simulink model "NonLinearMF"  (R2017a)
settings: Solver=ode5  StartTime=0.0  StopTime=30  FixedStep=0.01  RelTol=1e-3
values from neighbouring files (symbols this model uses):
  b10 = 6.05e-3    (= 0.00605)    [FurutaConstants.m]
  b20 = 5.52e-04    (= 0.000552)    [FurutaConstants.m]
  g0 = 9.81    [FurutaConstants.m]
  I1z0 = 3.7365e-3    (= 0.0037365)    [FurutaConstants.m]
  I2x0 = 0.2927e-3    (= 0.0002927)    [FurutaConstants.m]
  I2y0 = 0.2937e-3    (= 0.0002937)    [FurutaConstants.m]
  I2z0 = 0.0051e-3    (= 5.1e-06)    [FurutaConstants.m]
  Ixz20 = -0.0131e-3    (= -1.31e-05)    [FurutaConstants.m]
  K = [0 0 0 1]*(inv(M))*Phi    [Ackermanns.m]    (also in FurutaConstants.m = place(A,B,poles1))
  kt0 = 0.122326    [FurutaConstants.m]
  L10 = 230.45e-3    (= 0.23045)    [FurutaConstants.m]
  l10 = -56.69e-3    (= -0.05669)    [FurutaConstants.m]
  l20 = 58.18e-3    (= 0.05818)    [FurutaConstants.m]
  m10 = 0.36233    [FurutaConstants.m]
  m20 = 0.04948    [FurutaConstants.m]
  Rm0 = 12.38    [FurutaConstants.m]
  theta1o = 0    [FurutaConstants.m]
  theta2o = 14*pi/180    (= 0.244346095279)    [FurutaConstants.m]
settings Model: Creator=felip  LastModifiedBy=felip

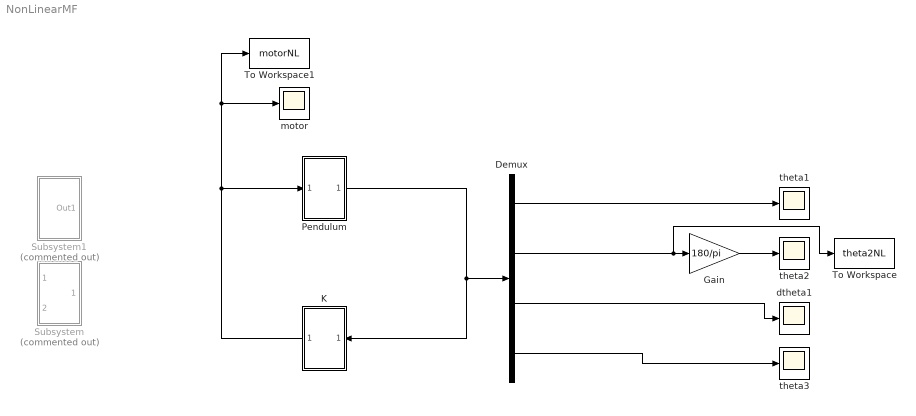
== system NonLinearMF ==
  Demux : Demux
  Gain : Gain  Gain=180/pi
  K : Subsystem
  Pendulum : Subsystem
  Subsystem : Subsystem  Commented=on
  Subsystem1 : Subsystem  Commented=on
  To Workspace : ToWorkspace  VariableName=theta2NL  SaveFormat=Timeseries  SampleTime=-1
  To Workspace1 : ToWorkspace  VariableName=motorNL  SaveFormat=Timeseries  SampleTime=-1
  dtheta1 : Scope
  "motor " : Scope
  theta1 : Scope
  theta2 : Scope
  theta3 : Scope
  wires:
  Pendulum/1(Out1) -> K/1(In1), Demux/1
  Demux/2 -> To Workspace/1, Gain/1
  Demux/1 -> theta1/1
  Demux/3 -> dtheta1/1
  Gain/1 -> theta2/1
  Demux/4 -> theta3/1
  K/1(Out1) -> Pendulum/1(In1), "motor "/1, To Workspace1/1

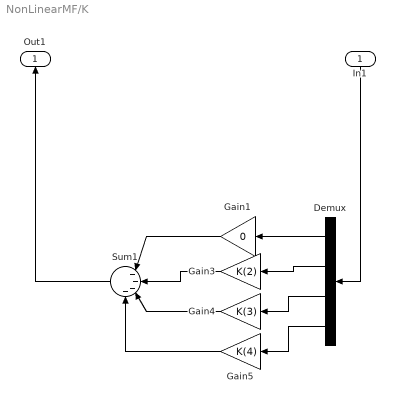
== system NonLinearMF/K ==
  In1 : Inport
  Demux : Demux
  Gain1 : Gain  Gain=0
  Gain3 : Gain  Gain=K(2)
  Gain4 : Gain  Gain=K(3)
  Gain5 : Gain  Gain=K(4)
  Sum1 : Sum  Inputs=|----
  Out1 : Outport
  wires:
  Demux/2 -> Gain3/1
  Demux/4 -> Gain5/1
  In1/1 -> Demux/1
  Gain4/1 -> Sum1/3
  Demux/3 -> Gain4/1
  Gain1/1 -> Sum1/1
  Gain5/1 -> Sum1/4
  Demux/1 -> Gain1/1
  Sum1/1 -> Out1/1
  Gain3/1 -> Sum1/2

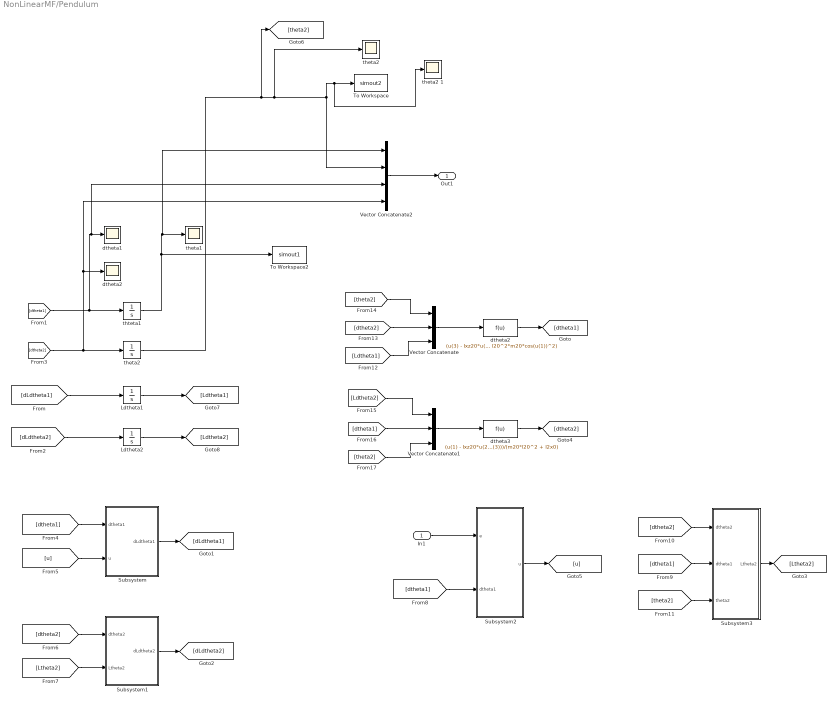
== system NonLinearMF/Pendulum ==
  In1 : Inport
  Ldtheta1 : Integrator
  Ldtheta2 : Integrator
  Subsystem : Subsystem
  Subsystem1 : Subsystem
  Subsystem2 : Subsystem
  Subsystem3 : Subsystem
  To Workspace : ToWorkspace  VariableName=simout2  SaveFormat=Timeseries  SampleTime=-1
  To Workspace2 : ToWorkspace  VariableName=simout1  SaveFormat=Timeseries  SampleTime=-1
  Vector Concatenate : Concatenate  NumInputs=3
  Vector Concatenate1 : Concatenate  NumInputs=3
  Vector Concatenate2 : Concatenate  NumInputs=4
  dtheta1 : Scope
  dtheta2 : Fcn  Expr=(u(3) - Ixz20*u(2)*cos(u(1)) + L10*u(2)*l20*m20*cos(u(1)))/(I2y0 + I1z0 + L10^2*m20 + l10^2*m10 + l20^2*m20 - I2y0*cos(u(1))^2 + I2z0*cos(u(1))^2 - l20^2*m20*cos(u(1))^2)
  "dtheta2 " : Scope
  dtheta3 : Fcn  Expr=(u(1) - Ixz20*u(2)*cos(u(3)) + L10*u(2)*l20*m20*cos(u(3)))/(m20*l20^2 + I2x0)
  theta1 : Scope
  theta2 : Integrator  InitialCondition=theta2o
  "theta2 " : Scope
  theta2 1 : Scope
  thteta1 : Integrator  InitialCondition=theta1o
  Out1 : Outport
  wires:
  In1/1 -> Subsystem2/1(e)
  Vector Concatenate2/1 -> Out1/1
  dtheta2/1 -> [dtheta1]
  [dtheta1] -> thteta1/1, Vector Concatenate2/3, dtheta1/1
  Subsystem1/1(dLdtheta2) -> [dLdtheta2]
  Vector Concatenate1/1 -> dtheta3/1
  [Ltheta2] -> Subsystem1/2(Ltheta2)
  Vector Concatenate/1 -> dtheta2/1
  [dtheta2] -> Vector Concatenate2/4, "dtheta2 "/1, theta2/1
  [dtheta1] -> Subsystem2/2(dtheta1)
  [theta2] -> Vector Concatenate1/3
  [dtheta2] -> Vector Concatenate/2
  [dLdtheta2] -> Ldtheta2/1
  [dLdtheta1] -> Ldtheta1/1
  Subsystem3/1("Ltheta2 ") -> [Ltheta2]
  Ldtheta1/1 -> [Ldtheta1]
  [theta2] -> Vector Concatenate/1
  Subsystem/1(dLdtheta1) -> [dLdtheta1]
  Ldtheta2/1 -> [Ldtheta2]
  [Ldtheta2] -> Vector Concatenate1/1
  thteta1/1 -> Vector Concatenate2/1, theta1/1, To Workspace2/1
  [dtheta1] -> Subsystem/1(dtheta1)
  [dtheta2] -> Subsystem1/1(dtheta2)
  Subsystem2/1("u ") -> [u]
  [theta2] -> Subsystem3/3(theta2)
  [dtheta1] -> Vector Concatenate1/2
  [dtheta1] -> Subsystem3/2(dtheta1)
  [Ldtheta1] -> Vector Concatenate/3
  [u] -> Subsystem/2(u)
  [dtheta2] -> Subsystem3/1(dtheta2)
  theta2/1 -> [theta2], Vector Concatenate2/2, theta2 1/1, To Workspace/1, "theta2 "/1
  dtheta3/1 -> [dtheta2]

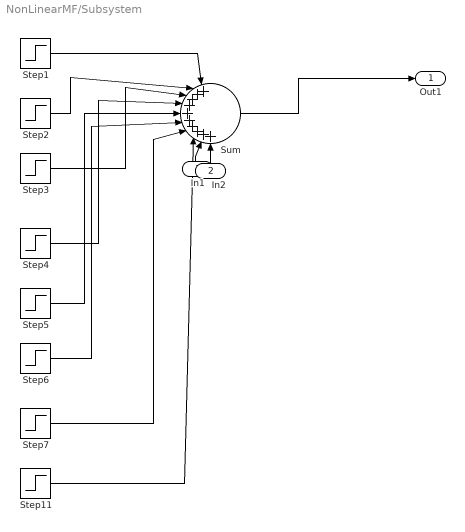
== system NonLinearMF/Subsystem ==
  In1 : Inport
  In2 : Inport  Port=2
  Step1 : Step  Time=10  After=12  SampleTime=0
  Step11 : Step  Time=14.68  After=-24  SampleTime=0
  Step2 : Step  Time=11.74  After=-24  SampleTime=0
  Step3 : Step  Time=12.28  After=24  SampleTime=0
  Step4 : Step  Time=12.76  After=-24  SampleTime=0
  Step5 : Step  Time=13.23  After=24  SampleTime=0
  Step6 : Step  Time=13.76  After=-24  SampleTime=0
  Step7 : Step  Time=14.23  After=24  SampleTime=0
  Sum : Sum  Inputs=|++++++++++
  Out1 : Outport
  wires:
  In2/1 -> Sum/10
  In1/1 -> Sum/9
  Step1/1 -> Sum/1
  Step4/1 -> Sum/4
  Step6/1 -> Sum/6
  Step2/1 -> Sum/2
  Step7/1 -> Sum/7
  Step3/1 -> Sum/3
  Step5/1 -> Sum/5
  Step11/1 -> Sum/8
  Sum/1 -> Out1/1

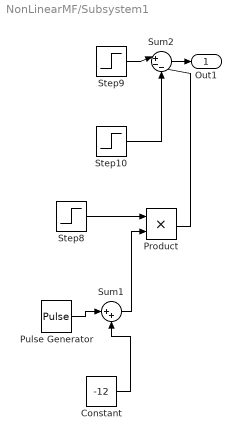
== system NonLinearMF/Subsystem1 ==
  Constant : Constant  Value=-12
  Product : Product
  Pulse Generator : DiscretePulseGenerator  PulseType=Time based  Amplitude=24  Period=1  PulseWidth=50
  Step10 : Step  Time=13.74  After=12  SampleTime=0
  Step8 : Step  Time=13.74  SampleTime=0
  Step9 : Step  Time=12  After=12  SampleTime=0
  Sum1 : Sum  Inputs=|++
  Sum2 : Sum  Inputs=|+--
  Out1 : Outport
  wires:
  Sum2/1 -> Out1/1
  Pulse Generator/1 -> Sum1/1
  Constant/1 -> Sum1/2
  Step8/1 -> Product/1
  Step10/1 -> Sum2/3
  Sum1/1 -> Product/2
  Step9/1 -> Sum2/1
  Product/1 -> Sum2/2

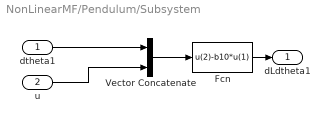
== system NonLinearMF/Pendulum/Subsystem ==
  dtheta1 : Inport
  u : Inport  Port=2
  Fcn : Fcn  Expr=u(2)-b10*u(1)
  Vector Concatenate : Concatenate
  dLdtheta1 : Outport
  wires:
  Fcn/1 -> dLdtheta1/1
  dtheta1/1 -> Vector Concatenate/1
  Vector Concatenate/1 -> Fcn/1
  u/1 -> Vector Concatenate/2

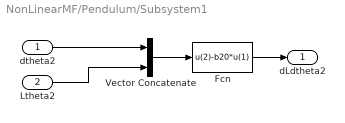
== system NonLinearMF/Pendulum/Subsystem1 ==
  dtheta2 : Inport
  Ltheta2 : Inport  Port=2
  Fcn : Fcn  Expr=u(2)-b20*u(1)
  Vector Concatenate : Concatenate
  dLdtheta2 : Outport
  wires:
  Fcn/1 -> dLdtheta2/1
  dtheta2/1 -> Vector Concatenate/1
  Vector Concatenate/1 -> Fcn/1
  Ltheta2/1 -> Vector Concatenate/2

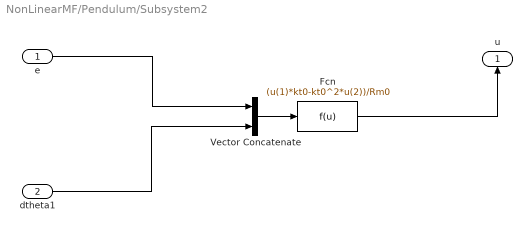
== system NonLinearMF/Pendulum/Subsystem2 ==
  e : Inport
  dtheta1 : Inport  Port=2
  Fcn : Fcn  Expr=(u(1)*kt0-kt0^2*u(2))/Rm0
  Vector Concatenate : Concatenate
  "u " : Outport
  wires:
  Fcn/1 -> "u "/1
  dtheta1/1 -> Vector Concatenate/2
  Vector Concatenate/1 -> Fcn/1
  e/1 -> Vector Concatenate/1

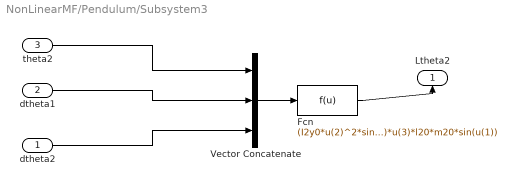
== system NonLinearMF/Pendulum/Subsystem3 ==
  dtheta2 : Inport
  dtheta1 : Inport  Port=2
  theta2 : Inport  Port=3
  Fcn : Fcn  Expr=(I2y0*u(2)^2*sin(2*u(1)))/2 - (I2z0*u(2)^2*sin(2*u(1)))/2 - Ixz20*u(2)*u(3)*sin(u(1)) + g0*l20*m20*sin(u(1)) + (u(2)^2*l20^2*m20*sin(2*u(1)))/2 + L10*u(2)*u(3)*l20*m20*sin(u(1))
  Vector Concatenate : Concatenate  NumInputs=3
  "Ltheta2 " : Outport
  wires:
  Fcn/1 -> "Ltheta2 "/1
  Vector Concatenate/1 -> Fcn/1
  dtheta2/1 -> Vector Concatenate/3
  dtheta1/1 -> Vector Concatenate/2
  theta2/1 -> Vector Concatenate/1
